simulink model "nonLinear"  (R2020b)
settings: Solver=ode15s  StartTime=0.0  StopTime=10  RelTol=1e-3
values from neighbouring files (symbols this model uses):
  A = [0 1 0;di11*mbg 0 0;di21*mbg 0 0]    [InitialParameters.m]
  B = [0;di12*km/R;di22*km/R]    [InitialParameters.m]
  C = eye(size(A))    [InitialParameters.m]
  D = zeros(size(C,1),size(B,2))    [InitialParameters.m]
  K = place(A,B,Vp)    [InitialParameters.m]
  Umax = 18    [InitialParameters.m]
settings Model: Creator=wildc  LastModifiedBy=clint
settings DataIOCC: ExternalInput=[t, u, x]  ReturnWorkspaceOutputs=off
settings DebuggingCC: AlgebraicLoopMsg=none  ArtificialAlgebraicLoopMsg=none

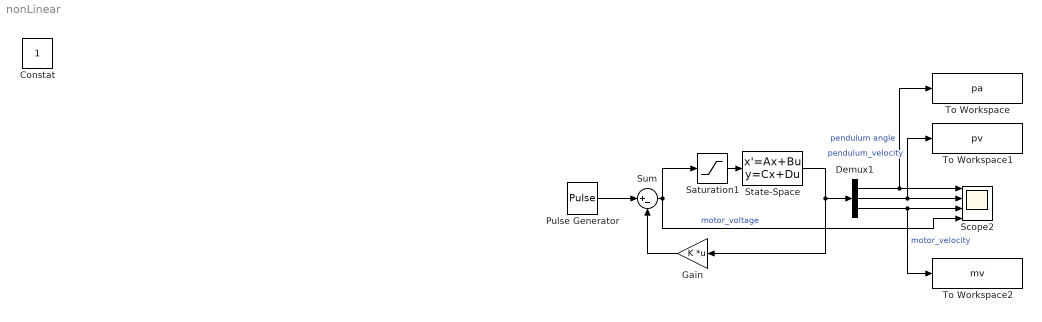
== system nonLinear ==
  Demux1 : Demux  Outputs=3
  Gain : Gain  Gain=K  Multiplication=Matrix(K*u)
  Pulse Generator : DiscretePulseGenerator  PulseType=Time based  Period=2.5  PulseWidth=5
  Saturation1 : Saturate  UpperLimit=Umax  LowerLimit=-Umax
  Scope2 : Scope  NumInputPorts=4
  State-Space : StateSpace  A=A  B=B  C=C  D=D  InitialCondition=[-.01 0 0]
  Sum : Sum  Inputs=|+-
  To Workspace : ToWorkspace  VariableName=pa  SampleTime=-1
  To Workspace1 : ToWorkspace  VariableName=pv  SampleTime=-1
  To Workspace2 : ToWorkspace  VariableName=mv  SampleTime=-1
  Constat : Constant  IOType=siggen
  wires:
  Demux1/1 -> To Workspace/1, Scope2/1  "pendulum angle"
  Demux1/2 -> To Workspace1/1, Scope2/2  "pendulum_velocity"
  Demux1/3 -> To Workspace2/1, Scope2/3  "motor_velocity"
  Saturation1/1 -> State-Space/1
  State-Space/1 -> Gain/1, Demux1/1
  Gain/1 -> Sum/2
  Sum/1 -> Scope2/4, Saturation1/1  "motor_voltage"
  Pulse Generator/1 -> Sum/1
